simulink library "powerlib"  (Simulink 6.0)
settings: Solver=ode45  SolverMode=SingleTasking  StartTime=0.0  StopTime=10.0  RelTol=1e-3
undefined symbols (not defined in the file or in its folder): com, ctrl1, Da, DiscIntNeverNeededParam, dtha, etat, FA, find_system, Ha, j, Ka, Ki, Kv, q0, Rground, sel, st_a, st_b, st_c, sta, stb, stc, T1, T2, T3, T4
libraries: powerlib_models x30, powerlib x25, simulink_extras x6, powerlib_extras x3, simulink x2
(part 5 of 7)

== system powerlib/Measurements ==
  note: ____ E x t r a s __________________________
  "  Extra Library " : Subsystem
      settings: OpenFcn=|
      | sys=sprintf('%s\n%s','powerlib_extras/Discrete','Measurements');
      | load_system('powerlib_extras');open_system(sys)
      mask Display: disp(['Discrete Measurements'])
  "  Extra Library 1" : Subsystem
      settings: OpenFcn=|
      | sys=sprintf('%s','powerlib_extras/Measurements');
      | load_system('powerlib_extras');open_system(sys)
      mask Display: disp(['Continuous Measurements'])
  "  Extra Library 2" : Subsystem
      settings: OpenFcn=|
      | sys=sprintf('%s\n%s','powerlib_extras/Phasor','Library');
      | load_system('powerlib_extras');open_system(sys)
      mask Display: disp(['Phasor Measurements'])
  Current Measurement : Subsystem  mask(Current Measurement){PhasorSimulation=off, OutputType=Complex, PSBequivalent=0}
      mask prompts: PhasorSimulation "Phasor simulation"; OutputType "Output signal :"; PSBequivalent "Equivalent circuit"
      mask help: Ideal current measurement.
      mask init:
      | block = gcb;
      | powericon('psbloadfunction',block,'Measurement Block','Initialize');
      | powericon('MeasurementBlockInit',block);
      settings: CopyFcn=powericon('psbloadfunction',gcb,'Measurement Block','UpdateGotoTag');
      settings: PreSaveFcn=|
      | if strcmp('inactive',get_param(gcb,'linkstatus'));
      | 
      | set_param(gcb,'Linkstatus','restore')
      | end
      mask Help: web(psbhelp);
      mask StyleString: checkbox,popup(Complex|Real-Imag|Magnitude-Angle|Magnitude),edit
  Impedance Measurement : PMComponent  PhysicalDomain=powersysdomain  LeftPortType=p1  RightPortType=p1  LConnTagsString=+|-  mask(Impedance Measurement){Factor=1}
      mask prompts: Factor "Multiplication factor"
      mask help: Measure the impedance between two nodes of a circuit as a function of the frequency. Use the Powergui block to display the impedance calculation.
      mask Help: web(psbhelp);
      mask Display: disp('Z')
  Multimeter : Subsystem  StopFcn=|  mask(MultimeterPSB){PhasorSimulation=off, OutputType=Complex, sel=1, L=1, Gain=0, yselected={}, PSBOutputType=1, PSBequivalent=0, AxesSetting=[0,0.1,-100,100], Display=0, SavedBlockNames=-11}
      | % This code will output Multimeter results in a plot when the simulation stops
      |                                                                               
      | powericon('psbsignals');
      mask prompts: PhasorSimulation "Phasor simulation"; OutputType "Output signal"; sel "output selection"; L "vector length"; yselected "yout identifier"; PSBOutputType "Output type [1=PSB  0=simulink output]"; PSBequivalent "Equivalent circuit"; AxesSetting "Axes"; Display "Display Window"
      mask init:
      | block = gcb;
      | powericon('psbloadfunction',block,'Measurement Block','Initialize');
      | powericon('MeasurementBlockInit',block);
      | NBS = length(sel);
      | NormalMode = [1:NBS];
      | NormalSignalLength = NBS;
      | switch OutputType
      | case {1,4}
      |     PhasorMode = [1:NBS];
      |     PhasorSignalLength = NBS;
      | case {2,3}
      |     for k=1:NBS;
      |         PhasorMode = [k,k+NBS];
      |     end
      |     PhasorSignalLength = 2*NBS;
      | end
      | if PhasorSimulation
      |     SelectionMode = PhasorMode;
      | 	SignalLength = PhasorSignalLength;
      | else
      |     SelectionMode = NormalMode;
      | 	SignalLength = NormalSignalLength;
      | end
      settings: CopyFcn=powericon('psbloadfunction',gcb,'Measurement Block','UpdateGotoTag');  OpenFcn=psbmultimeter(gcb,'PM')
      settings: PreSaveFcn=|
      | if strcmp('inactive',get_param(gcb,'linkstatus'));
      | 
      | set_param(gcb,'Linkstatus','restore');
      | set_param(gcb,'PSBequivalent','0');
      | end
      mask Help: web(psbhelp)
      mask StyleString: checkbox,popup(Complex|Real_Imag|Magnitude-angle|Magnitude),edit,edit,edit,edit,edit,edit,edit,edit,edit
      mask Display:
      | plot(0,0,100,100,[10,10,90,90,10],[90,10,10,90,90]);
      | disp(length(sel)*(sum(abs(Gain))>0))
  Three-Phase V-I Measurement : Subsystem  mask(Three-Phase VI Measurement){VoltageMeasurement=phase-to-ground, SetLabelV=off, LabelV=Vabc, Vpu=off, Vbase=500e3, CurrentMeasurement=yes, SetLabelI=off, LabelI=Iabc, Ipu=off, Pbase=100e6, OutputType=Complex, PhasorSimulation=off, PSBequivalent=0}
      mask prompts: VoltageMeasurement "Voltage measurement"; SetLabelV "Use a label"; LabelV "Signal label  (use a From block to collect signal)"; Vpu "Voltage  in pu"; Vbase "Base voltage (Vrms phase-phase) :"; CurrentMeasurement "Current measurement"; SetLabelI "Use a label"; LabelI "Signal label  (use a From block to collect signal)"; Ipu "Currents in pu"; Pbase "Base power ( VA 3 phase)"; OutputType "Output signal :"; PhasorSimulation "Phasor simulation"; PSBequivalent "Equivalent circuit"
      mask help:
      | This block is used to measure three-phase voltages and currents in a circuit. When connected in series with a  three-phase element, it return the three phase-to-ground voltages and line currents.
      |
      | The block can output the voltages and currents in per unit values or in volts and amperes. Check the appropriate boxes if you want to output the voltages and currents  in pu
      mask init:
      | block = gcb;
      | [Kv,Ki,SelectionModeV,SelectionModeI,SignalLength]=powericon('ThreePhaseVIMeasurementParam',Vpu,Ipu,Vbase,Pbase,OutputType,PhasorSimulation);
      | powericon('psbcallbacks',block,'Three-phase VI measurements',4);
      | powericon('psbloadfunction',block,'3-Phase VI Measurement','Initialize');
      | powericon('MeasurementBlockInit',block);
      settings: CopyFcn=powericon('psbloadfunction',gcb,'3-Phase VI Measurement','UpdateGotoTag');
      settings: PreSaveFcn=|
      | try
      | set_param(gcb,'Linkstatus','restore')
      | end
      mask Help: web(psbhelp)
      mask StyleString: popup(no|phase-to-ground|phase-to-phase),checkbox,edit,checkbox,edit,popup(no|yes),checkbox,edit,checkbox,edit,popup(Complex|Real-Imag|Magnitude-Angle|Magnitude),checkbox,edit
      mask CallbackString: powericon('psbcallbacks',gcb,'Three-phase VI measurements',2);|powericon('psbcallbacks',gcb,'Three-phase VI measurements',2);||powericon('psbcallbacks',gcb,'Three-phase VI measurements',2);||powericon('psbcallbacks',gcb,'Three-phase VI measurements',2);|powericon('psbcallbacks',gcb,'Three-phase VI measurements',2);||powericon('psbcallbacks',gcb,'Three-phase VI measurements',4);||||
  Voltage Measurement : Subsystem  mask(Voltage Measurement){PhasorSimulation=off, OutputType=Complex, PSBequivalent=0}
      mask prompts: PhasorSimulation "Phasor simulation"; OutputType "Output signal :"; PSBequivalent "Equivalent circuit"
      mask help: Ideal voltage measurement.
      mask init:
      | block = gcb;
      | powericon('psbloadfunction',block,'Measurement Block','Initialize');
      | powericon('MeasurementBlockInit',block);
      settings: CopyFcn=powericon('psbloadfunction',gcb,'Measurement Block','UpdateGotoTag');
      settings: PreSaveFcn=|
      | if strcmp('inactive',get_param(gcb,'linkstatus'));
      | 
      | set_param(gcb,'Linkstatus','restore')
      | end
      mask Help: web(psbhelp);
      mask StyleString: checkbox,popup(Complex|Real-Imag|Magnitude-Angle|Magnitude),edit

== system powerlib/Phasor Elements ==
  note: ____ F l e x i b l e A C T r a n s m i s s i o n S y s t e m s ( F A C T S ) _______
  Static Var Compensator : Subsystem  LoadFcn=find_system(gcs,'FollowLinks', 'on', 'LookUnderMasks', 'all');  mask(Static Var Compensator (Phasor Type)){mode=Var control (Fixed susceptance Bref), Vnom=500e3, Qnom=[200e6  -100e6], Pbase=200e6, Vref=1.0, Xs=0.03, Kp_Ki=[0  300], Bref=0.5, Tm=8e-3, Td=4e-3}
      mask prompts: mode "Mode of operation"; Vnom "Nominal voltage (Vrms Ph-Ph):"; Qnom "Reactive power limits [Qc(var>0)  Ql(var<0)]:"; Pbase "Three-phase base power Pbase (VA):"; Vref "Reference voltage Vref  (pu):"; Xs "Droop Xs (pu/Pbase):"; Kp_Ki "Voltage regulator [Kp(puB/puV)  Ki(puB/puV/s)]:"; Bref "Bref  for var control mode (pu/Pbase):"; Tm "Time constant of voltage measurement system Tm (s):"; Td "Average time delay due to thyristor valves firing Td (s):"
      mask help:
      | This block implements a  phasor model of a three-phase, three-wire Static Var Compensator (SVC).
      |
      | The B output signal (SVC susceptance in pu/Pbase)  is the output of the voltage regulator or the reference susceptance Bref in var control mode.
      | The Vm output is the measured positive-sequence voltage (pu).
      mask init:
      | Qc_nom=Qnom(1);
      | Ql_nom=Qnom(2);
      | Bmax=Qc_nom/Pbase;
      | Bmin=Ql_nom/Pbase;
      | Vbase=Vnom/sqrt(3)*sqrt(2);
      | Ibase=Pbase/Vnom/sqrt(3)*sqrt(2);
      | Kp=Kp_Ki(1);
      | Ki=Kp_Ki(2);;
      settings: CloseFcn=%3phaseVImeasurement
      mask Help: web(psbhelp)
      mask StyleString: popup(Voltage regulation|Var control (Fixed susceptance Bref)),edit,edit,edit,edit,edit,edit,edit,edit,edit
      mask CallbackString: powericon('psbcallbacks',gcb,'SVCblock');|||||||||

== system powerlib/Power Electronics ==
  note: ____ E x t r a s ____________________________________________________
  note: ____ D e v i c e s __________________________________________________
  "  Extra Library " : Subsystem
      settings: OpenFcn=sys=sprintf('%s\n%s','powerlib_extras/Discrete ','Control Blocks');powerlib_extras([],[],[],'load');open_system(sys)
      mask Display: disp(['Discrete Control blocks'])
  "  Extra Library 1" : Subsystem
      settings: OpenFcn=sys=sprintf('%s\n%s','powerlib_extras/Control ','Blocks');powerlib_extras([],[],[],'load');open_system(sys)
      mask Display: disp(['Control blocks'])
  Detailed Thyristor : Subsystem  mask(Detailed Thyristor){Ron=0.001, Lon=0, Vf=0.8, IL=0.1, Tq=100e-6, IC=0, Rs=500, Cs=250e-9, Measurements=on}
      mask prompts: Ron "Resistance Ron (Ohms) :"; Lon "Inductance Lon (H) :"; Vf "Forward voltage Vf (V) :"; IL "Latching current Il (A) :"; Tq "Turn-off time Tq (s) :"; IC "Initial current Ic (A) :"; Rs "Snubber resistance Rs (Ohms) :"; Cs "Snubber capacitance Cs (F) :"; Measurements "Show measurement port"
      mask help:
      | Detailed model of Thyristor in parallel with a series RC snubber circuit. In on-state the Thyristor model  has an internal resistance (Ron) and inductance (Lon).  For most applications the internal inductance should be set to zero. In off-state the Detailed Thyristor  as an impedance.
      |
      | Best accuracy is achieved when Tq is larger than the simulation step size.
      mask init:
      | block = gcb;
      | s=powericon('PowerSwitch',Rs,Cs);
      | powericon('psbcallbacks',block,'measurement output');
      | powericon('psbloadfunction',block,'gotofrom','Initialize');
      settings: CopyFcn=powericon('psbloadfunction',gcb,'gotofrom','UpdateGotoTag');
      mask Help: web(psbhelp);
      mask CallbackString: ||||||||powericon('psbcallbacks',gcb,'measurement output');
      mask Display: plot(-140,-140,140,140,2*[-30,-30,0,-30,-30,-55]+25,(2*[20,0,20,41,20,20]+8),[0,0]+25,(2*[0,40]+8),2*[37.5,0]+25,(2*[20,20]+8),2*[10,10,0]+25,(1*[-15,6,20]+12),s*[-65,-65,-20,-20,40,40,85,85,85,40,40,-20,-20],s*[48,-20,-20,-10,-10,-20,-20,48,-20,-20,-30,-30,-20])
  Diode : Subsystem  mask(Diode){Ron=0.001, Lon=0, Vf=0.8, IC=0, Rs=500, Cs=250e-9, Measurements=off}
      mask prompts: Ron "Resistance Ron (Ohms) :"; Lon "Inductance Lon (H) :"; Vf "Forward voltage Vf (V) :"; IC "Initial current Ic (A) :"; Rs "Snubber resistance Rs (Ohms) :"; Cs "Snubber capacitance Cs (F) :"; Measurements "Show measurement port"
      mask help: Implements a diode in parallel with a series RC snubber circuit. In on-state the Diode model has an internal resistance (Ron) and inductance (Lon). For most applications the internal inductance should be set to zero. The Diode impedance is infinite in off-state mode.
      mask init:
      | block = gcb;
      | s=powericon('PowerSwitch',Rs,Cs);
      | powericon('psbcallbacks',block,'measurement output');
      | powericon('psbloadfunction',block,'from','Initialize');
      settings: CopyFcn=powericon('psbloadfunction',gcb,'from','UpdateGotoTag');
      mask Help: web(psbhelp);
      mask CallbackString: ||||||powericon('psbcallbacks',gcb,'measurement output');
      mask Display: plot(-75,-50,100,150,[-15,-15,43,-15,-15,-75],[50,8,50,92,50,50],[43,43],[8,94],[100,43],[50,50],s*[-65,-65,-20,-20,40,40,85,85,85,40,40,-20,-20],s*[50,-20,-20,-10,-10,-20,-20,50,-20,-20,-30,-30,-20])
  Gto : Subsystem  mask(Gto){Ron=0.001, Lon=1e-6, Vf=1, Tf=10e-6, Tt=20e-6, IC=0, Rs=1e5, Cs=inf, Measurements=on}
      mask prompts: Ron "Resistance Ron (Ohms) :"; Lon "Inductance Lon (H) :"; Vf "Forward voltage Vf (V) :"; Tf "Current 10% fall time Tf (s) :"; Tt "Current tail time Tt (s) :"; IC "Initial current Ic (A) :"; Rs "Snubber resistance Rs (Ohms) :"; Cs "Snubber capacitance Cs (F) :"; Measurements "Show Measurement port"
      mask help:
      | Implements a GTO thyristor in parallel with a series RC snubber circuit.
      | In on-state the GTO model has internal resistance (Ron) and inductance (Lon).
      | In off-state the GTO model has infinite impedance.
      |
      | The internal inductance cannot be set to zero.Discretization of the GTO is
      | available only through the Universal Bridge block.
      mask init:
      | block = gcb;
      | s=powericon('PowerSwitch',Rs,Cs);
      | powericon('psbcallbacks',block,'measurement output');
      | powericon('psbloadfunction',block,'gotofrom','Initialize');
      settings: CopyFcn=powericon('psbloadfunction',gcb,'gotofrom','UpdateGotoTag');
      mask Help: web(psbhelp);
      mask CallbackString: ||||||||powericon('psbcallbacks',gcb,'measurement output');
      mask Display: plot(-140,-140,140,140,2*[-30,-30,0,-30,-30,-60]+25,(2*[20,0,20,41,20,20]+8),[0,0]+25,(2*[0,40]+8),2*[35,0]+25,(2*[20,20]+8),2*[10,10,0]+25,(2*[-15,6,20]+8),[20,0]+35,[-8,-8],s*[-75,-75,-20,-20,20,20,75,75,75,20,20,-20,-20],s*([78,0,0,10,10,0,0,78,0,0,-10,-10,0]-30))
  IGBT : Subsystem  mask(IGBT){Ron=0.001, Lon=1e-6, Vf=1, Tf=1e-6, Tt=2e-6, IC=0, Rs=1e5, Cs=inf, Measurements=on}
      mask prompts: Ron "Resistance Ron (Ohms) :"; Lon "Inductance Lon (H) :"; Vf "Forward voltage Vf (V) :"; Tf "Current 10% fall time Tf (s) :"; Tt "Current tail time Tt (s):"; IC "Initial current Ic (A) :"; Rs "Snubber resistance Rs (Ohms) :"; Cs "Snubber capacitance Cs (F) :"; Measurements "Show measurement port"
      mask help:
      | Implements an IGBT device  in parallel with a series RC snubber circuit. In on-state the IGBT model has internal resistance (Ron) and inductance (Lon). In off-state the IGBT model has infinite impedance. The internal inductance cannot be set to zero.
      | Discretization of the IGBT is available only through the Universal Bridge block.
      mask init:
      | block = gcb;
      | s=powericon('PowerSwitch',Rs,Cs);
      | powericon('psbcallbacks',block,'measurement output');
      | powericon('psbloadfunction',block,'gotofrom','Initialize');
      settings: CopyFcn=powericon('psbloadfunction',gcbh,'gotofrom','UpdateGotoTag');
      mask Help: web(psbhelp);
      mask CallbackString: ||||||||powericon('psbcallbacks',gcb,'measurement output');
      mask Display: plot(-15,0,115,100,[82,82,18],[16,35,35],[3,19,35,18,80,60,76,97],[65,65,45,45,45,45,65,65],[81,83,72,81]-7,[65,58,60,65],s*([-75,-75,-20,-20,20,20,75,75,75,20,20,-20,-20]*.45+50),s*([0,50,50,60,60,50,50,0,50,50,40,40,50]*.4+65))
  Ideal Switch : Subsystem  mask(Ideal Switch){Ron=0.001, Lon=0, IC=0, Rs=1e5, Cs=inf, Measurements=on}
      mask prompts: Ron "Internal resistance Ron (Ohms) :"; Lon "Inductance Lon (H) :"; IC "Initial state (0 for 'open', 1 for 'closed') :"; Rs "Snubber resistance Rs (Ohms) :"; Cs "Snubber capacitance Cs (F) :"; Measurements "Show measurement port"
      mask help:
      | Switch controlled by a gate signal, in parallel with a series RC snubber circuit. In on-state the Switch model has an internal resistance (Ron) . In off-state this internal resistance is infinite. The internal resistance must be greather than zero.
      |
      | The switch model is on-state when the gate signal (g) is set to 1.
      mask init:
      | block = gcb;
      | s=powericon('PowerSwitch',Rs,Cs);
      | powericon('psbcallbacks',block,'measurement output');
      | powericon('psbloadfunction',block,'gotofrom','Initialize');
      settings: CopyFcn=powericon('psbloadfunction',gcb,'gotofrom','UpdateGotoTag');
      mask Help: web(psbhelp);
      mask CallbackString: |||||powericon('psbcallbacks',gcb,'measurement output');
      mask Display: plot(-120,-40,120,140,[-100,-30,5],[50,50,95],[20,100],[50,50],s*[-75,-75,-20,-20,20,20,75,75,75,20,20,-20,-20],s*[50,0,0,10,10,0,0,50,0,0,-10,-10,0])
  Mosfet : Subsystem  mask(Mosfet){Ron=0.001, Lon=1e-6, Rd=.001, IC=0, Rs=1e5, Cs=inf, Measurements=on}
      mask prompts: Ron "Resistance Ron (Ohms) :"; Lon "Inductance Lon (H) :"; Rd "Internal diode resistance Rd  (Ohms) :"; IC "Initial current Ic (A) :"; Rs "Snubber resistance Rs (Ohms) :"; Cs "Snubber capacitance Cs (F) :"; Measurements "Show measurement port"
      mask help:
      | MOSFET in parallel with a series RC snubber circuit. In on-state the MOSFET model has internal resistance (Ron) and inductance (Lon). In off-state the MOSFET model has infinite impedance. The internal inductance cannot be set to zero.
      | Discretization of the MOSFET is available only through the Universal Bridge block.
      mask init:
      | block = gcb;
      | s=powericon('PowerSwitch',Rs,Cs);
      | powericon('psbcallbacks',block,'measurement output');
      | powericon('psbloadfunction',block,'gotofrom','Initialize');
      settings: CopyFcn=powericon('psbloadfunction',gcb,'gotofrom','UpdateGotoTag');
      mask Help: web(psbhelp);
      mask CallbackString: ||||||powericon('psbcallbacks',gcb,'measurement output');
      mask Display: plot(-160,-140,140,140,2*[33,23,28,28,10,10,35,55,55,90,55,55,35,35,35,35,0]-100,(2*[28,28,28,50,50,75,75,65,75,75,75,85,75,65,85,75,75]-100),2*[50,39,45,38,52,45,45,65,65,60,70,65,65,82,82]-100,(2*[28,28,28,39,39,28,50,50,28,28,28,28,50,50,75]-100),2*[70,70,23]-100,(2*[7,20,20]-100),s*[-50,-50,-30,-30,10,10,32,32,32,10,10,-30,-30],s*([45,80,80,85,85,80,80,45,80,80,75,75,80]+5))
  Three-Level Bridge : Subsystem  mask(Three-Level Bridge){Arms=3, SnubberResistance=1e5, SbubberCapacitance=inf, Device=GTO / Diodes, Ron=1e-3, ForwardVoltages=[  0  0  ], Measurements=None}
      mask prompts: Arms "Number of bridge arms:"; SnubberResistance "Snubber resistance Rs (Ohms)"; SbubberCapacitance "Snubber capacitance Cs (F)"; Device "Power Electronic device"; Ron "Internal resistance Ron (Ohms)"; ForwardVoltages "Forward voltages  [ Device Vf(V) , Diode Vfd(V)]"
      mask help: This block implements a three-level bridge of selected forced-commutated power electronics devices. Series RC snubber circuits are connected in parallel with each switch device. Press Help for suggested snubber values when the model is discretized.
      mask init:
      | block = gcb;
      | powericon('psbloadfunction',block,'configurable bridge','Initialize');
      | if Device==4
      |     switch Arms
      |     case 1
      |         selection1 = [1,2,4];
      |         selection2 = [1,3,4];
      |     case 2
      |         selection1 = [1,2,4,5,6,8];
      |         selection2 = [1,3,4,5,7,8];
      |     case 3
      |         selection1 = [1,2,4,5,6,8,9,10,12];
      |         selection2 = [1,3,4,5,7,8,9,11,12];
      |     end
      | else
      |     selection1 = [1:4*Arms];
      |     selection2 = [1:4*Arms];
      | end
      | %
      | powericon('ThreeLevelBridgeCback',block,'device configuration');
      | powericon('ThreeLevelBridgeCback',block,'BridgeArms');
      settings: CopyFcn=powericon('psbloadfunction',gcb,'configurable bridge','UpdateGotoTag');
      mask Help: web(psbhelp);
      mask StyleString: popup(1|2|3),edit,edit,popup(GTO / Diodes|MOSFET / Diodes|IGBT / Diodes|Ideal Switches),edit,edit,popup(None|All device currents|Phase-to-Neutral and DC voltages|All voltages and currents)
      mask CallbackString: powericon('ThreeLevelBridgeCback',gcb,'BridgeArms');|||powericon('ThreeLevelBridgeCback',gcb,'device configuration');|||
      mask Display: plot(0,0,100,100,[40 28 52 40 24 52 40 40],[40 60 60 40 40 40 40 10],[40,40],[90,60],[16 28 40],[25,25,40],[21.6 35.2],[25,40],[65 57 73 65 57 73 65 65],[54 42 42 54 54 54 54 66],[40 65 65],[24 24 42],[65 65 40],[66,76,76]);
  Thyristor : Subsystem  mask(Thyristor){Ron=0.001, Lon=0, Vf=0.8, IC=0, Rs=500, Cs=250e-9, Measurements=on}
      mask prompts: Ron "Resistance Ron (Ohms) :"; Lon "Inductance Lon (H) :"; Vf "Forward voltage Vf (V) :"; IC "Initial current Ic (A) :"; Rs "Snubber resistance Rs (Ohms) :"; Cs "Snubber capacitance Cs (F) :"; Measurements "Show measurement port"
      mask help: Thyristor in parallel with a series RC snubber circuit. In on-state the Thyristor model has an internal resistance (Ron) and inductance (Lon). For most applications the internal inductance should be set to zero. In off-state the Thyristor as an infinite impedance.
      mask init:
      | block = gcb;
      | s=powericon('PowerSwitch',Rs,Cs);
      | powericon('psbcallbacks',block,'measurement output');
      | powericon('psbloadfunction',block,'gotofrom','Initialize');
      settings: CopyFcn=powericon('psbloadfunction',gcb,'gotofrom','UpdateGotoTag');
      mask Help: web(psbhelp);
      mask CallbackString: ||||||powericon('psbcallbacks',gcb,'measurement output');
      mask Display: plot(-140,-140,140,140,2*[-30,-30,0,-30,-30,-55]+25,(2*[20,0,20,41,20,20]+8),[0,0]+25,(2*[0,40]+8),2*[37.5,0]+25,(2*[20,20]+8),2*[10,10,0]+25,(1*[-15,6,20]+12),s*[-65,-65,-20,-20,40,40,85,85,85,40,40,-20,-20],s*[48,-20,-20,-10,-10,-20,-20,48,-20,-20,-30,-30,-20])
  Universal Bridge : Subsystem  mask(Universal Bridge){Arms=3, SnubberResistance=1e5, SnubberCapacitance=inf, Device=Thyristors, Ron=1e-3, Lon=0, ForwardVoltages=[  0  0  ], ForwardVoltage=0, GTOparameters=[ 10e-6 , 20e-6 ], IGBTparameters=[ 1e-6 , 2e-6 ], Measurements=None}
      mask prompts: Arms "Number of bridge arms:"; SnubberResistance "Snubber resistance Rs (Ohms)"; SnubberCapacitance "Snubber capacitance Cs (F)"; Device "Power Electronic device"; Ron "Ron (Ohms)"; Lon "Lon (H)"; ForwardVoltages "Forward voltages  [ Device Vf(V) , Diode Vfd(V)]"; ForwardVoltage "Forward voltage Vf (V)"; GTOparameters "[  Tf (s) , Tt (s)  ]"; IGBTparameters "[  Tf (s) , Tt (s)  ]"
      mask help: This block implement a bridge of selected power electronics devices. Series RC snubber circuits are connected in parallel with each switch device. Press Help for suggested snubber values when the model is discretized. For most applications the internal inductance Lon of diodes and thyristors should be set to zero
      mask init:
      | block = gcb;
      | powericon('TwoLevelBridgeCback',block,'device configuration');
      | powericon('TwoLevelBridgeCback',block,'BridgeArms');
      | powericon('psbloadfunction',block,'configurable bridge','Initialize');
      settings: CopyFcn=powericon('psbloadfunction',gcb,'configurable bridge','UpdateGotoTag');
      mask Help: web(psbhelp);
      mask StyleString: popup(1|2|3),edit,edit,popup(Diodes|Thyristors|GTO / Diodes|MOSFET / Diodes|IGBT / Diodes|Ideal Switches),edit,edit,edit,edit,edit,edit,popup(None|Device voltages|Device currents|UAB UBC UCA UDC voltages|All voltages and currents)
      mask CallbackString: powericon('TwoLevelBridgeCback',gcb,'BridgeArms');|||powericon('TwoLevelBridgeCback',gcb,'device configuration');|||||||
      mask Display: plot(0,0,100,100,[50,30,70,50,30,70,50,50],[60,30,30,60,60,60,60,90],[50,50],[10,30],[20,35,50],[75,75,60]);

== system powerlib/powergui ==
  Subsystem : Subsystem

== system powerlib/Electrical Sources/AC Current Source ==
  ACCurrentSource : PMComponent  PhysicalDomain=powersysdomain  LeftPortType=p1  RightPortType=p1  LConnTagsString=a  RConnTagsString=__new0
      mask Type: InnerPowersysBlock
  Source : Sin  Amplitude=Amplitude  Frequency=2*pi*Frequency  Phase=Phase*pi/180  SampleTime=SampleTime
  - : PMIOPort  Port=1  Side=Left
  + : PMIOPort  Orientation=left  Port=2  Side=Right
  tag scope: LibraryTag=global
  wires:
  Source/1 -> [LibraryTag]
  connections:
  -/RConn1 -- ACCurrentSource/LConn1
  ACCurrentSource/RConn1 -- +/RConn1

== system powerlib/Electrical Sources/AC Voltage Source ==
  ACVoltageSource : PMComponent  PhysicalDomain=powersysdomain  LeftPortType=p1  RightPortType=p1  LConnTagsString=a  RConnTagsString=__new0
      mask Type: InnerPowersysBlock
  Source : Sin  Amplitude=Amplitude  Frequency=2*pi*Frequency  Phase=Phase*pi/180  SampleTime=SampleTime
  - : PMIOPort  Port=1  Side=Left
  + : PMIOPort  Orientation=left  Port=2  Side=Right
  tag scope: LibraryTag=global
  wires:
  Source/1 -> [LibraryTag]
  connections:
  -/RConn1 -- ACVoltageSource/LConn1
  +/RConn1 -- ACVoltageSource/RConn1

== system powerlib/Electrical Sources/Controlled Current Source ==
  s : Inport  Port=1  LatchInput=off
  ControlledCurrentSource : PMComponent  PhysicalDomain=powersysdomain  LeftPortType=p1  RightPortType=p1  LConnTagsString=a  RConnTagsString=__new0
      mask Type: InnerPowersysBlock
  - : PMIOPort  Port=1  Side=Left
  + : PMIOPort  Orientation=left  Port=2  Side=Right
  tag scope: LibraryTag=global
  wires:
  s/1 -> [LibraryTag]
  connections:
  ControlledCurrentSource/RConn1 -- +/RConn1
  -/RConn1 -- ControlledCurrentSource/LConn1

== system powerlib/Electrical Sources/Controlled Voltage Source ==
  s : Inport  Port=1  LatchInput=off
  ControlledVoltageSource : PMComponent  PhysicalDomain=powersysdomain  LeftPortType=p1  RightPortType=p1  LConnTagsString=a  RConnTagsString=__new0
      mask Type: InnerPowersysBlock
  - : PMIOPort  Port=1  Side=Left
  + : PMIOPort  Orientation=left  Port=2  Side=Right
  tag scope: LibraryTag=global
  wires:
  s/1 -> [LibraryTag]
  connections:
  ControlledVoltageSource/RConn1 -- +/RConn1
  -/RConn1 -- ControlledVoltageSource/LConn1

== system powerlib/Electrical Sources/DC Voltage Source ==
  DCVoltageSource : PMComponent  PhysicalDomain=powersysdomain  LeftPortType=p1  RightPortType=p1  LConnTagsString=a  RConnTagsString=__new0
      mask Type: InnerPowersysBlock
  Source : Constant  Value=Amplitude
  - : PMIOPort  Port=1  Side=Left
  + : PMIOPort  Orientation=left  Port=2  Side=Right
  tag scope: LibraryTag=global
  wires:
  Source/1 -> [LibraryTag]
  connections:
  -/RConn1 -- DCVoltageSource/LConn1
  +/RConn1 -- DCVoltageSource/RConn1

== system powerlib/Electrical Sources/Three-Phase Programmable Voltage Source ==
  Source : powerlib_models/Continuous/3_Phase_Prog_Source
  ThreePhasePrgSrcBlk : PMComponent  PhysicalDomain=powersysdomain  LeftPortType=p1  RightPortType=p1  LConnTagsString=N  RConnTagsString=A|B|C
      mask Type: InnerPowersysBlock
  N : PMIOPort  Port=1  Side=Left
  A : PMIOPort  Orientation=left  Port=2  Side=Right
  B : PMIOPort  Orientation=left  Port=3  Side=Right
  C : PMIOPort  Orientation=left  Port=4  Side=Right
  tag scope: LibraryTag=global
  wires:
  Source/1 -> [LibraryTag]
  connections:
  A/RConn1 -- ThreePhasePrgSrcBlk/RConn1
  N/RConn1 -- ThreePhasePrgSrcBlk/LConn1
  B/RConn1 -- ThreePhasePrgSrcBlk/RConn2
  C/RConn1 -- ThreePhasePrgSrcBlk/RConn3

== system powerlib/Electrical Sources/Three-Phase Source ==
  Source : powerlib_models/Sources/ThreePhaseSource
  ThreePhaseSourceBlk : PMComponent  PhysicalDomain=powersysdomain  LeftPortType=p1  RightPortType=p1  LConnTagsString=N  RConnTagsString=A|B|C
      mask Type: InnerPowersysBlock
  A : PMIOPort  Orientation=left  Port=1  Side=Right
  B : PMIOPort  Orientation=left  Port=2  Side=Right
  C : PMIOPort  Orientation=left  Port=3  Side=Right
  tag scope: LibraryTag=global
  wires:
  Source/1 -> [LibraryTag]
  connections:
  A/RConn1 -- ThreePhaseSourceBlk/RConn1
  B/RConn1 -- ThreePhaseSourceBlk/RConn2
  C/RConn1 -- ThreePhaseSourceBlk/RConn3

== system powerlib/Elements/Breaker ==
  c : Inport  Port=1  LatchInput=off
  Breaker : PMComponent  PhysicalDomain=powersysdomain  LeftPortType=p1  RightPortType=p1  LConnTagsString=a  RConnTagsString=__new0
      mask Type: InnerPowersysBlock
  C4 : Constant  Value=com
  Data Type  Conversion : DataTypeConversion  OutDataTypeMode=double  SaturateOnIntegerOverflow=on  RndMeth=Zero
  Switch3 : Switch  Threshold=0.5  ZeroCross=off  InputSameDT=on
  Timer : powerlib_extras/Control  Blocks/Timer  t=SwitchingTimes  e=switchings
  1 : PMIOPort  Port=1  Side=Left
  2 : PMIOPort  Orientation=left  Port=2  Side=Right
  tag scope: LibraryTag=global
  wires:
  Switch3/1 -> [LibraryTag]
  C4/1 -> Switch3/2
  Timer/1 -> Switch3/3
  c/1 -> Data Type  Conversion/1
  Data Type  Conversion/1 -> Switch3/1
  connections:
  2/RConn1 -- Breaker/RConn1
  1/RConn1 -- Breaker/LConn1

== system powerlib/Elements/Distributed Parameters Line ==
  DistributedParametersLine : PMComponent  PhysicalDomain=powersysdomain  LeftPortType=p1  RightPortType=p1  LConnTagsString=1|2|3  RConnTagsString=1|2|3
      mask Type: InnerPowersysBlock
  Source : powerlib_models/Continuous/distributed_param_line  nphase=Phases  f=Frequency  ri=Resistance  li=Inductance  ci=Capacitance  long=Length  V1_init=x1  V2_init=x2  I1_init=x3  I2_init=x4  time_init=x5
  i1 : PMIOPort  Port=1  Side=Left
  i2 : PMIOPort  Port=2  Side=Left
  i3 : PMIOPort  Port=3  Side=Left
  o1 : PMIOPort  Orientation=left  Port=4  Side=Right
  o2 : PMIOPort  Orientation=left  Port=5  Side=Right
  o3 : PMIOPort  Orientation=left  Port=6  Side=Right
  tag scope: LibraryTag=global
  wires:
  [LibraryTag] -> Source/1
  Source/1 -> [LibraryTag]
  connections:
  i1/RConn1 -- DistributedParametersLine/LConn1
  o1/RConn1 -- DistributedParametersLine/RConn1
  i2/RConn1 -- DistributedParametersLine/LConn2
  o2/RConn1 -- DistributedParametersLine/RConn2
  i3/RConn1 -- DistributedParametersLine/LConn3
  o3/RConn1 -- DistributedParametersLine/RConn3

== system powerlib/Elements/Multi-Winding Transformer ==
  NWindingsTransformer : PMComponent  PhysicalDomain=powersysdomain  LeftPortType=p1  RightPortType=p1  LConnTagsString=1|2  RConnTagsString=1|2|3|4|5|6
      mask Type: InnerPowersysBlock
  1+ : PMIOPort  Port=1  Side=Left
  1 : PMIOPort  Port=2  Side=Left
  +2 : PMIOPort  Orientation=left  Port=3  Side=Right
  2 : PMIOPort  Orientation=left  Port=4  Side=Right
  +3 : PMIOPort  Orientation=left  Port=5  Side=Right
  3 : PMIOPort  Orientation=left  Port=6  Side=Right
  +4 : PMIOPort  Orientation=left  Port=7  Side=Right
  4 : PMIOPort  Orientation=left  Port=8  Side=Right
  connections:
  1+/RConn1 -- NWindingsTransformer/LConn1
  1/RConn1 -- NWindingsTransformer/LConn2
  NWindingsTransformer/RConn1 -- +2/RConn1
  NWindingsTransformer/RConn2 -- 2/RConn1
  NWindingsTransformer/RConn3 -- +3/RConn1
  NWindingsTransformer/RConn4 -- 3/RConn1
  NWindingsTransformer/RConn5 -- +4/RConn1
  NWindingsTransformer/RConn6 -- 4/RConn1

== system powerlib/Elements/Saturable Transformer ==
  Goto2 : Terminator
  SaturableTransformer : PMComponent  PhysicalDomain=powersysdomain  LeftPortType=p1  RightPortType=p1  LConnTagsString=A|B  RConnTagsString=1|2|3|4
      mask Type: InnerPowersysBlock
  Source : powerlib_models/Continuous/saturable_transformer  SaturationFlux=SaturationFlux  SaturationCurrent=SaturationCurrent  InitialFlux=InitialFlux
  A : PMIOPort  Port=1  Side=Left
  B : PMIOPort  Port=2  Side=Left
  1 : PMIOPort  Orientation=left  Port=3  Side=Right
  2 : PMIOPort  Orientation=left  Port=4  Side=Right
  3 : PMIOPort  Orientation=left  Port=5  Side=Right
  4 : PMIOPort  Orientation=left  Port=6  Side=Right
  tag scope: LibraryTag=global
  wires:
  [LibraryTag] -> Source/1
  Source/1 -> [LibraryTag]
  Source/2 -> Goto2/1
  connections:
  B/RConn1 -- SaturableTransformer/LConn2
  A/RConn1 -- SaturableTransformer/LConn1
  SaturableTransformer/RConn1 -- 1/RConn1
  SaturableTransformer/RConn2 -- 2/RConn1
  SaturableTransformer/RConn3 -- 3/RConn1
  SaturableTransformer/RConn4 -- 4/RConn1

== system powerlib/Elements/Surge Arrester ==
  Source : powerlib_models/Continuous/surge_arrester  uref=ProtectionVoltage  n=Columns  iref=ReferenceCurrent  param1=Segment1  param2=Segment2  param3=Segment3  BreakLoop=1
  SurgeArrester : PMComponent  PhysicalDomain=powersysdomain  LeftPortType=p1  RightPortType=p1  LConnTagsString=a  RConnTagsString=__new0
      mask Type: InnerPowersysBlock
  1 : PMIOPort  Port=1  Side=Left
  2 : PMIOPort  Orientation=left  Port=2  Side=Right
  tag scope: LibraryTag=global
  wires:
  Source/1 -> [LibraryTag]
  [LibraryTag] -> Source/1
  connections:
  1/RConn1 -- SurgeArrester/LConn1
  2/RConn1 -- SurgeArrester/RConn1

== system powerlib/Elements/Three-Phase Dynamic Load ==
  3-PhaseDynamicLoad : PMComponent  PhysicalDomain=powersysdomain  LeftPortType=p1  RightPortType=p1  LConnTagsString=A|B  RConnTagsString=C
      mask Type: InnerPowersysBlock
  Measurement list : Subsystem
  PQ : Ground
  Source : powerlib_models/Continuous/Dynamic_Load
  A : PMIOPort  Port=1  Side=Left
  B : PMIOPort  Port=2  Side=Left
  C : PMIOPort  Orientation=left  Port=3  Side=Left
  m : Outport  InitialOutput=[0,0,0]
  tag scope: LibraryTag=global
  wires:
  Measurement list/1(Out1) -> m/1
  Source/1 -> [LibraryTag]
  [LibraryTag] -> Source/1
  PQ/1 -> Source/2
  Source/2 -> Measurement list/1(In1)
  connections:
  A/RConn1 -- 3-PhaseDynamicLoad/LConn1
  B/RConn1 -- 3-PhaseDynamicLoad/LConn2
  C/RConn1 -- 3-PhaseDynamicLoad/RConn1

== system powerlib/Elements/Three-Phase Transformer (Three Windings) ==
  Three-PhaseTransformer : PMComponent  PhysicalDomain=powersysdomain  LeftPortType=p1  RightPortType=p1  LConnTagsString=A|B|C  RConnTagsString=a2|b2|c2|a3|b3|c3
      mask Type: InnerPowersysBlock
  A : PMIOPort  Port=1  Side=Left
  B : PMIOPort  Port=2  Side=Left
  C : PMIOPort  Port=3  Side=Left
  a2 : PMIOPort  Orientation=left  Port=4  Side=Right
  b2 : PMIOPort  Orientation=left  Port=5  Side=Right
  c2 : PMIOPort  Orientation=left  Port=6  Side=Right
  a3 : PMIOPort  Orientation=left  Port=7  Side=Right
  b3 : PMIOPort  Orientation=left  Port=8  Side=Right
  c3 : PMIOPort  Orientation=left  Port=9  Side=Right
  connections:
  A/RConn1 -- Three-PhaseTransformer/LConn1
  B/RConn1 -- Three-PhaseTransformer/LConn2
  C/RConn1 -- Three-PhaseTransformer/LConn3
  Three-PhaseTransformer/RConn6 -- c3/RConn1
  Three-PhaseTransformer/RConn5 -- b3/RConn1
  Three-PhaseTransformer/RConn4 -- a3/RConn1
  c2/RConn1 -- Three-PhaseTransformer/RConn3
  Three-PhaseTransformer/RConn2 -- b2/RConn1
  Three-PhaseTransformer/RConn1 -- a2/RConn1

== system powerlib/Elements/Three-Phase Transformer (Two Windings) ==
  Three-PhaseTransformer : PMComponent  PhysicalDomain=powersysdomain  LeftPortType=p1  RightPortType=p1  LConnTagsString=A|B|C  RConnTagsString=a|b|c
      mask Type: InnerPowersysBlock
  A : PMIOPort  Port=1  Side=Left
  B : PMIOPort  Port=2  Side=Left
  C : PMIOPort  Port=3  Side=Left
  a : PMIOPort  Orientation=left  Port=4  Side=Right
  b : PMIOPort  Orientation=left  Port=5  Side=Right
  c : PMIOPort  Orientation=left  Port=6  Side=Right
  connections:
  a/RConn1 -- Three-PhaseTransformer/RConn1
  b/RConn1 -- Three-PhaseTransformer/RConn2
  c/RConn1 -- Three-PhaseTransformer/RConn3
  A/RConn1 -- Three-PhaseTransformer/LConn1
  B/RConn1 -- Three-PhaseTransformer/LConn2
  C/RConn1 -- Three-PhaseTransformer/LConn3

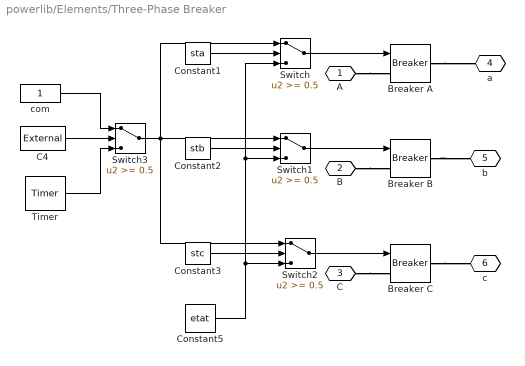
== system powerlib/Elements/Three-Phase Breaker ==
  Breaker A : powerlib/Elements/Breaker  BreakerResistance=BreakerResistance  InitialState=etat  SnubberResistance=SnubberResistance  SnubberCapacitance=SnubberCapacitance  SwitchingTimes="[ 1/60  5/60 ]"  External=on  Measurements=None
  Breaker B : powerlib/Elements/Breaker  BreakerResistance=BreakerResistance  InitialState=etat  SnubberResistance=SnubberResistance  SnubberCapacitance=SnubberCapacitance  SwitchingTimes="[ 1/60  5/60 ]"  External=on  Measurements=None
  Breaker C : powerlib/Elements/Breaker  BreakerResistance=BreakerResistance  InitialState=etat  SnubberResistance=SnubberResistance  SnubberCapacitance=SnubberCapacitance  SwitchingTimes="[ 1/60  5/60 ]"  External=on  Measurements=None
  C4 : Constant  Value=External
  Constant1 : Constant  Value=sta
  Constant2 : Constant  Value=stb
  Constant3 : Constant  Value=stc
  Constant5 : Constant  Value=etat
  Switch{,1..3} (4 alike) : Switch  Threshold=0.5  ZeroCross=off  InputSameDT=on
  Timer : powerlib_extras/Control  Blocks/Timer  t=sw_times  e=switchings
  com : Constant
  A : PMIOPort  Port=1  Side=Left
  B : PMIOPort  Port=2  Side=Left
  C : PMIOPort  Port=3  Side=Left
  a : PMIOPort  Orientation=left  Port=4  Side=Right
  b : PMIOPort  Orientation=left  Port=5  Side=Right
  c : PMIOPort  Orientation=left  Port=6  Side=Right
  wires:
  Constant5/1 -> Switch2/3, Switch1/3, Switch/3
  Timer/1 -> Switch3/3
  com/1 -> Switch3/1
  C4/1 -> Switch3/2
  Switch1/1 -> Breaker B/1
  Constant2/1 -> Switch1/2
  Switch2/1 -> Breaker C/1
  Constant3/1 -> Switch2/2
  Switch/1 -> Breaker A/1
  Constant1/1 -> Switch/2
  Switch3/1 -> Switch2/1, Switch/1, Switch1/1
  connections:
  Breaker C/RConn1 -- c/RConn1
  Breaker B/RConn1 -- b/RConn1
  Breaker A/RConn1 -- a/RConn1
  C/RConn1 -- Breaker C/LConn1
  B/RConn1 -- Breaker B/LConn1
  A/RConn1 -- Breaker A/LConn1

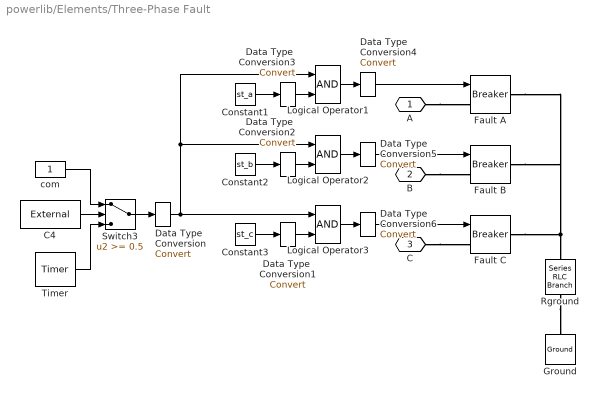
== system powerlib/Elements/Three-Phase Fault ==
  C4 : Constant  Value=External
  Constant1 : Constant  Value=st_a
  Constant2 : Constant  Value=st_b
  Constant3 : Constant  Value=st_c
  Data Type  Conversion{,1..3} (4 alike) : DataTypeConversion  OutDataTypeMode=boolean  SaturateOnIntegerOverflow=on  RndMeth=Zero
  Data Type  Conversion4 : DataTypeConversion  OutDataTypeMode=double  SaturateOnIntegerOverflow=on  RndMeth=Zero
  Data Type  Conversion5 : DataTypeConversion  OutDataTypeMode=double  SaturateOnIntegerOverflow=on  RndMeth=Zero
  Data Type  Conversion6 : DataTypeConversion  OutDataTypeMode=double  SaturateOnIntegerOverflow=on  RndMeth=Zero
  Fault A : powerlib/Elements/Breaker  BreakerResistance=FaultResistance  InitialState=init_a  SnubberResistance=SnubberResistance  SnubberCapacitance=SnubberCapacitance  SwitchingTimes="[ 1/60  5/60 ]"  External=on  Measurements=None
  Fault B : powerlib/Elements/Breaker  BreakerResistance=FaultResistance  InitialState=init_b  SnubberResistance=SnubberResistance  SnubberCapacitance=SnubberCapacitance  SwitchingTimes="[ 1/60  5/60 ]"  External=on  Measurements=None
  Fault C : powerlib/Elements/Breaker  BreakerResistance=FaultResistance  InitialState=init_c  SnubberResistance=SnubberResistance  SnubberCapacitance=SnubberCapacitance  SwitchingTimes="[ 1/60  5/60 ]"  External=on  Measurements=None
  Ground : powerlib/Elements/Ground  Orientation=down  PhysicalDomain=powersysdomain  SubClassName=unknown  LeftPortType=p1  RightPortType=p1  LConnTagsString=a  RConnTagsString=__newr0
  Logical Operator1 : Logic
  Logical Operator2 : Logic
  Logical Operator3 : Logic
  Rground : powerlib/Elements/Series RLC Branch  Orientation=down  PhysicalDomain=powersysdomain  SubClassName=unknown  LeftPortType=p1  RightPortType=p1  LConnTagsString=__new0  RConnTagsString=__new0  Resistance=Rground  Inductance=0  Capacitance=inf  Measurements=None
  Switch3 : Switch  Threshold=0.5  ZeroCross=off  InputSameDT=on
  Timer : powerlib_extras/Control  Blocks/Timer  t=SwitchTimes  e=SwitchStatus
  com : Constant
  A : PMIOPort  Port=1  Side=Left
  B : PMIOPort  Port=2  Side=Left
  C : PMIOPort  Port=3  Side=Left
  wires:
  Data Type  Conversion6/1 -> Fault C/1
  Data Type  Conversion5/1 -> Fault B/1
  Data Type  Conversion4/1 -> Fault A/1
  Logical Operator3/1 -> Data Type  Conversion6/1
  Logical Operator2/1 -> Data Type  Conversion5/1
  Logical Operator1/1 -> Data Type  Conversion4/1
  Data Type  Conversion3/1 -> Logical Operator1/2
  Constant1/1 -> Data Type  Conversion3/1
  Data Type  Conversion2/1 -> Logical Operator2/2
  Constant2/1 -> Data Type  Conversion2/1
  Data Type  Conversion1/1 -> Logical Operator3/2
  Constant3/1 -> Data Type  Conversion1/1
  Data Type  Conversion/1 -> Logical Operator1/1, Logical Operator2/1, Logical Operator3/1
  Switch3/1 -> Data Type  Conversion/1
  C4/1 -> Switch3/2
  Timer/1 -> Switch3/3
  com/1 -> Switch3/1
  connections:
  Fault C/RConn1 -- Rground/LConn1 -- Fault B/RConn1 -- Fault A/RConn1
  C/RConn1 -- Fault C/LConn1
  B/RConn1 -- Fault B/LConn1
  A/RConn1 -- Fault A/LConn1
  Rground/RConn1 -- Ground/LConn1

== system powerlib/Elements/Three-Phase Transformer 12 Terminals ==
  T1 : powerlib/Elements/Linear Transformer  PhysicalDomain=powersysdomain  SubClassName=unknown  LeftPortType=p1  RightPortType=p1  LConnTagsString=a|b  RConnTagsString=A|B  NominalPower=[pnom fnom]  winding1=Winding1  winding2=Winding2  ThreeWindings=off  winding3=[60e3 0.005 0.02]  RmLm=RmXm  Measurements=None
  T2 : powerlib/Elements/Linear Transformer  PhysicalDomain=powersysdomain  SubClassName=unknown  LeftPortType=p1  RightPortType=p1  LConnTagsString=a|b  RConnTagsString=A|B  NominalPower=[pnom fnom]  winding1=Winding1  winding2=Winding2  ThreeWindings=off  winding3=[60e3 0.005 0.02]  RmLm=RmXm  Measurements=None
  T3 : powerlib/Elements/Linear Transformer  PhysicalDomain=powersysdomain  SubClassName=unknown  LeftPortType=p1  RightPortType=p1  LConnTagsString=a|b  RConnTagsString=A|B  NominalPower=[pnom fnom]  winding1=Winding1  winding2=Winding2  ThreeWindings=off  winding3=[60e3 0.005 0.02]  RmLm=RmXm  Measurements=None
  A1+ : PMIOPort  Port=1  Side=Left
  A1 : PMIOPort  Port=2  Side=Left
  B1+ : PMIOPort  Port=3  Side=Left
  B1 : PMIOPort  Port=4  Side=Left
  C1+ : PMIOPort  Port=5  Side=Left
  C1 : PMIOPort  Port=6  Side=Left
  A2+ : PMIOPort  Orientation=left  Port=7  Side=Right
  A2 : PMIOPort  Orientation=left  Port=8  Side=Right
  B2+ : PMIOPort  Orientation=left  Port=9  Side=Right
  B2 : PMIOPort  Orientation=left  Port=10  Side=Right
  C2+ : PMIOPort  Orientation=left  Port=11  Side=Right
  C2 : PMIOPort  Orientation=left  Port=12  Side=Right
  connections:
  T3/RConn2 -- C2/RConn1
  T3/RConn1 -- C2+/RConn1
  C1/RConn1 -- T3/LConn2
  C1+/RConn1 -- T3/LConn1
  T2/RConn2 -- B2/RConn1
  T2/RConn1 -- B2+/RConn1
  B1/RConn1 -- T2/LConn2
  B1+/RConn1 -- T2/LConn1
  T1/RConn2 -- A2/RConn1
  A1/RConn1 -- T1/LConn2
  T1/RConn1 -- A2+/RConn1
  A1+/RConn1 -- T1/LConn1

== system powerlib/Elements/Zigzag Phase-Shifting Transformer ==
  Three-PhaseTransformer : PMComponent  PhysicalDomain=powersysdomain  LeftPortType=p1  RightPortType=p1  LConnTagsString=1|2|3|4|5|6  RConnTagsString=a|b|c
      mask Type: InnerPowersysBlock
  A+ : PMIOPort  Port=1  Side=Left
  B+ : PMIOPort  Port=2  Side=Left
  C+ : PMIOPort  Port=3  Side=Left
  A- : PMIOPort  Port=4  Side=Left
  B- : PMIOPort  Port=5  Side=Left
  C- : PMIOPort  Port=6  Side=Left
  a3 : PMIOPort  Orientation=left  Port=7  Side=Right
  b3 : PMIOPort  Orientation=left  Port=8  Side=Right
  c3 : PMIOPort  Orientation=left  Port=9  Side=Right
  connections:
  A+/RConn1 -- Three-PhaseTransformer/LConn1
  B+/RConn1 -- Three-PhaseTransformer/LConn2
  C+/RConn1 -- Three-PhaseTransformer/LConn3
  A-/RConn1 -- Three-PhaseTransformer/LConn4
  B-/RConn1 -- Three-PhaseTransformer/LConn5
  C-/RConn1 -- Three-PhaseTransformer/LConn6
  Three-PhaseTransformer/RConn3 -- c3/RConn1
  b3/RConn1 -- Three-PhaseTransformer/RConn2
  a3/RConn1 -- Three-PhaseTransformer/RConn1

== system powerlib/Machines/Asynchronous Machine SI Units ==
  Tm : Inport  Orientation=left  Port=1  LatchInput=off
  ASM : PMComponent  PhysicalDomain=powersysdomain  LeftPortType=p1  RightPortType=p1  LConnTagsString=A|B|C  RConnTagsString=a|b|c
      mask Type: InnerPowersysBlock
  ASM_mechanics : powerlib_models/Continuous/ASM_mechanics  Orientation=left
  Measurement list : Subsystem
  Source : powerlib_models/Continuous/asynchronous_machine
  A : PMIOPort  Port=1  Side=Left
  B : PMIOPort  Port=2  Side=Left
  C : PMIOPort  Port=3  Side=Left
  a : PMIOPort  Orientation=left  Port=4  Side=Right
  b : PMIOPort  Orientation=left  Port=5  Side=Right
  c : PMIOPort  Orientation=left  Port=6  Side=Right
  m : Outport  InitialOutput=0
  tag scope: LibraryTag=global
  wires:
  Measurement list/1(Out1) -> m/1
  Tm/1 -> ASM_mechanics/1
  Source/3 -> ASM_mechanics/2
  Source/1 -> [LibraryTag]
  [LibraryTag] -> Source/1
  ASM_mechanics/2 -> Source/2
  Source/2 -> Measurement list/1(m_e)
  ASM_mechanics/1 -> Measurement list/2(m_m)
  connections:
  c/RConn1 -- ASM/RConn3
  ASM/RConn2 -- b/RConn1
  ASM/RConn1 -- a/RConn1
  C/RConn1 -- ASM/LConn3
  B/RConn1 -- ASM/LConn2
  A/RConn1 -- ASM/LConn1

== system powerlib/Machines/Asynchronous Machine pu Units ==
  Tm : Inport  Orientation=left  Port=1  LatchInput=off
  ASM : PMComponent  PhysicalDomain=powersysdomain  LeftPortType=p1  RightPortType=p1  LConnTagsString=A|B|C  RConnTagsString=a|b|c
      mask Type: InnerPowersysBlock
  ASM_mechanics : powerlib_models/Continuous/ASM_mechanics  Orientation=left
  Measurement list : Subsystem
  Source : powerlib_models/Continuous/asynchronous_machine
  A : PMIOPort  Port=1  Side=Left
  B : PMIOPort  Port=2  Side=Left
  C : PMIOPort  Port=3  Side=Left
  a : PMIOPort  Orientation=left  Port=4  Side=Right
  b : PMIOPort  Orientation=left  Port=5  Side=Right
  c : PMIOPort  Orientation=left  Port=6  Side=Right
  m : Outport  InitialOutput=0
  tag scope: LibraryTag=global
  wires:
  Measurement list/1(Out1) -> m/1
  [LibraryTag] -> Source/1
  Source/1 -> [LibraryTag]
  Source/3 -> ASM_mechanics/2
  ASM_mechanics/2 -> Source/2
  Tm/1 -> ASM_mechanics/1
  Source/2 -> Measurement list/1(m_e)
  ASM_mechanics/1 -> Measurement list/2(m_m)
  connections:
  C/RConn1 -- ASM/LConn3
  B/RConn1 -- ASM/LConn2
  A/RConn1 -- ASM/LConn1
  ASM/RConn1 -- a/RConn1
  ASM/RConn2 -- b/RConn1
  ASM/RConn3 -- c/RConn1

== system powerlib/Machines/DC Machine ==
  TL : Inport  Port=1  LatchInput=off
  FCEM : powerlib/Electrical Sources/Controlled Voltage Source  Description=source block  Orientation=up  Initialize=on  Amplitude=0  Phase=0  Frequency=0  Measurements=None
  Measurement list : Subsystem
  Mechanics : Subsystem
  Ra La : powerlib/Elements/Series RLC Branch  PhysicalDomain=powersysdomain  SubClassName=unknown  LeftPortType=p1  RightPortType=p1  LConnTagsString=__new0  RConnTagsString=__new0  Resistance=Ra  Inductance=La  Capacitance=inf  Measurements=None
  Rf  Lf : powerlib/Elements/Series RLC Branch  PhysicalDomain=powersysdomain  SubClassName=unknown  LeftPortType=p1  RightPortType=p1  LConnTagsString=__new0  RConnTagsString=__new0  Resistance=Rf  Inductance=Lf  Capacitance=inf  Measurements=None
  iA : powerlib/Measurements/Current Measurement  PhasorSimulation=off  OutputType=Magnitude  PSBequivalent=0
  iF : powerlib/Measurements/Current Measurement  PhasorSimulation=off  OutputType=Magnitude  PSBequivalent=0
  A+ : PMIOPort  Port=1  Side=Left
  A- : PMIOPort  Orientation=up  Port=2  Side=Right
  F+ : PMIOPort  Port=3  Side=Left
  F- : PMIOPort  Orientation=left  Port=4  Side=Right
  m : Outport
  wires:
  Mechanics/2(m) -> Measurement list/1(In1)
  TL/1 -> Mechanics/1(TL)
  iF/1 -> Mechanics/3(if)
  Mechanics/1(FCEM) -> FCEM/1
  iA/1 -> Mechanics/2(ia)
  Measurement list/1(Out1) -> m/1
  connections:
  F-/RConn1 -- Rf  Lf/RConn1
  A-/RConn1 -- FCEM/LConn1
  Rf  Lf/LConn1 -- iF/RConn1
  Ra La/LConn1 -- iA/RConn1
  FCEM/RConn1 -- Ra La/RConn1
  iF/LConn1 -- F+/RConn1
  iA/LConn1 -- A+/RConn1

== system powerlib/Machines/Discrete DC Machine ==
  TL : Inport  Port=1  LatchInput=off
  FCEM : powerlib/Electrical Sources/Controlled Voltage Source  Description=source block  Orientation=up  Initialize=on  Amplitude=0  Phase=0  Frequency=0  Measurements=None
  Measurement list : Subsystem
  Mechanics : Subsystem
  Ra La : powerlib/Elements/Series RLC Branch  PhysicalDomain=powersysdomain  SubClassName=unknown  LeftPortType=p1  RightPortType=p1  LConnTagsString=__new0  RConnTagsString=__new0  Resistance=Ra  Inductance=La  Capacitance=inf  Measurements=None
  Rf  Lf : powerlib/Elements/Series RLC Branch  PhysicalDomain=powersysdomain  SubClassName=unknown  LeftPortType=p1  RightPortType=p1  LConnTagsString=__new0  RConnTagsString=__new0  Resistance=Rf  Inductance=Lf  Capacitance=inf  Measurements=None
  iA : powerlib/Measurements/Current Measurement  PhasorSimulation=off  OutputType=Magnitude  PSBequivalent=0
  iF : powerlib/Measurements/Current Measurement  PhasorSimulation=off  OutputType=Magnitude  PSBequivalent=0
  A+ : PMIOPort  Port=1  Side=Left
  A- : PMIOPort  Orientation=up  Port=2  Side=Right
  F+ : PMIOPort  Port=3  Side=Left
  F- : PMIOPort  Orientation=left  Port=4  Side=Right
  m : Outport
  wires:
  iA/1 -> Mechanics/2(iA)
  Mechanics/2(FCEM) -> FCEM/1
  iF/1 -> Mechanics/3(iF)
  TL/1 -> Mechanics/1(TL)
  Mechanics/1(m) -> Measurement list/1(In1)
  Measurement list/1(Out1) -> m/1
  connections:
  FCEM/RConn1 -- Ra La/RConn1
  Ra La/LConn1 -- iA/RConn1
  Rf  Lf/LConn1 -- iF/RConn1
  iA/LConn1 -- A+/RConn1
  A-/RConn1 -- FCEM/LConn1
  iF/LConn1 -- F+/RConn1
  F-/RConn1 -- Rf  Lf/RConn1
